simulink model "animation"  (R2020a)
settings: Solver=VariableStepAuto  StartTime=0.0  StopTime=10.0  RelTol=1e-3
libraries: vrlib x3, robotcorelib x1, robotmaniplib x1
settings Model: Creator=BS-chen  LastModifiedBy=BS-chen

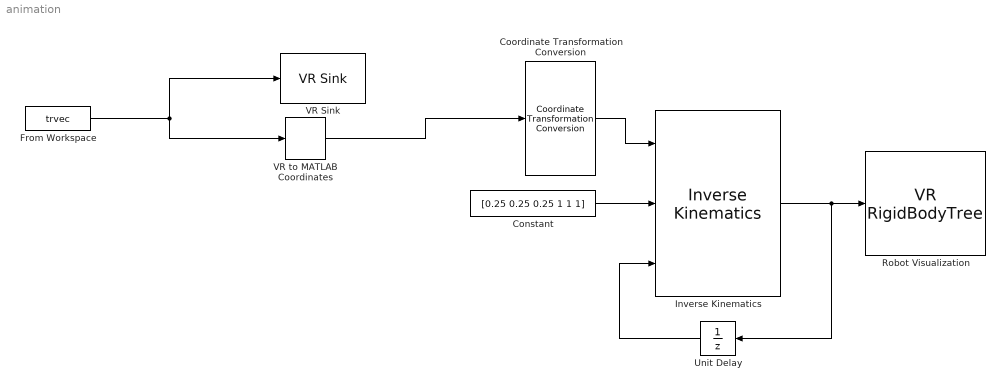
== system animation ==
  Constant : Constant  Value=[0.25 0.25 0.25 1 1 1]
  Coordinate Transformation Conversion : robotcorelib/Coordinate Transformation Conversion  InputRepresentation=Translation Vector  InputEulerSequence=ZYX  ShowTrVecInputPort=on  OutputRepresentation=Homogeneous Transformation  OutputEulerSequence=ZYX  ShowTrVecOutputPort=on  SimulateUsing=Interpreted execution
      settings: SourceProductBaseCode=NV,RO,RR
  From Workspace : FromWorkspace  VariableName=trvec
  Inverse Kinematics : robotmaniplib/Inverse Kinematics  RigidBodyTree=robot  EndEffector=body6  ShowInfo=off  SolverName=BFGS Gradient Projection  EnforceJointLimits=on  MaxIterations=40  MaxTime=10  GradientTolerance=1e-7  SolutionTolerance=1e-6  StepTolerance=1e-14  ErrorChangeTolerance=1e-12  UseErrorDamping=on  DampingBias=0.0025  SimulateUsing=Interpreted execution
  Robot Visualization : vrlib/VR RigidBodyTree  RBT=robot  useRBT=off  Ts=0.1  ForceViewerOpen=off
      settings: SourceProductBaseCode=SL
  Unit Delay : UnitDelay  InitialCondition=zeros(7,1)  SampleTime=-1  HasFrameUpgradeWarning=on
  VR Sink : vrlib/VR Sink  InstantiateOnLoad=on  SampleTime=-1  ViewEnable=on  RemoteChange=off  RemoteView=off  FieldsWritten=SetPoint.translation.3.1.1.double  WorldFileName=robot_scene.x3d  WorldDescription=Rigid Body Tree Visualization  AutoView=on  VideoDimensions=[]  AllowVariableSize=off
  VR to MATLAB Coordinates : vrlib/Utilities/VR to MATLAB Coordinates
      settings: SourceProductBaseCode=SL
  wires:
  Coordinate Transformation Conversion/1 -> Inverse Kinematics/1
  Unit Delay/1 -> Inverse Kinematics/3
  Inverse Kinematics/1 -> Unit Delay/1, Robot Visualization/1
  Constant/1 -> Inverse Kinematics/2
  From Workspace/1 -> VR to MATLAB Coordinates/1, VR Sink/1
  VR to MATLAB Coordinates/1 -> Coordinate Transformation Conversion/1
